simulink model "ex_pdcont"  (R2013a)
settings: Solver=ode1  StartTime=0.0  StopTime=inf  FixedStep=0.001  RelTol=1e-3
values from neighbouring files (symbols this model uses):
  kD = -0.399    [pdcont_data1.mat]    (also in pdcont_data2.mat = -0.022; pdcont_data3.mat = 0.261)
  kP = 7.075    [pdcont_data1.mat]    (also in pdcont_data2.mat; pdcont_data3.mat)
undefined symbols (not defined in the file or in its folder): HIL
libraries: quarc_library x3
settings Model: SimulationMode=external  ExtModeTrigDuration=500000  Creator=student  LastModifiedBy=student
settings SolverCC: PositivePriorityOrder=on
settings RTWCC: SystemTargetFile=quarc_win64.tlc  TemplateMakefile=quarc_default_tmf  Description=QUARC Win64 Target  ProcessScript=quarc_win64_make_rtw_hook
settings STFCustomTargetCC: TargetPreCompLibLocation=C:\PROGRA~3\QUARC\lib\2013a\win64\release  GeneratePreprocessorConditionals=Disable all  CombineOutputUpdateFcns=on  SystemTargetFile=quarc_win64.tlc
settings GRTTargetCC: TargetPreCompLibLocation=C:\PROGRA~3\QUARC\lib\2013a\win64\release  ParMdlRefBuildCompliant=off  CompOptLevelCompliant=off  ConcurrentExecutionCompliant=off  MatFileLogging=off  ExtMode=on  ExtModeMexFile=quarc_comm

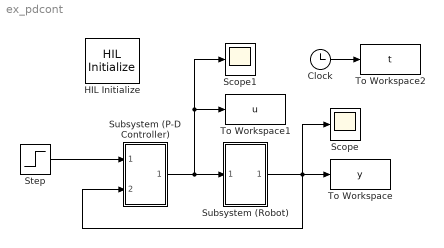
== system ex_pdcont ==
  Clock : Clock
  HIL Initialize : quarc_library/Data Acquisition/Generic/Configuration/HIL Initialize  Priority=-99  object_name=HIL-1  board_type=q8_usb  board_number=0  board_options=update_rate=normal;decimation=1  exclusive=off  active=off  hardware_clocks=[0:2]  clock_modes=[]  initial_clock_frequencies=[]  set_clock_params_at_start=off  set_clock_params_at_switch_in=off  set_clock_frequencies_at_start=off  set_clock_frequencies_at_switch_in=off  analog_input_channels=[0:7]  analog_input_maximums=5  analog_input_minimums=-5  set_analog_input_params_at_start=on  set_analog_input_params_at_switch_in=off  analog_output_channels=[0:7]  analog_output_maximums=10  analog_output_minimums=-10  initial_analog_outputs=[0]  final_analog_outputs=[0]  watchdog_analog_outputs=0  set_analog_output_params_at_start=on  set_analog_output_params_at_switch_in=off  set_analog_outputs_at_start=on  set_analog_outputs_at_switch_in=off  set_analog_outputs_at_terminate=on  set_analog_outputs_at_switch_out=off  set_analog_outputs_on_watchdog=off  digital_input_channels=[]  digital_output_channels=[]  digital_output_configuration=[]  initial_digital_outputs=[1]  final_digital_outputs=[1]  watchdog_digital_outputs=[1]  set_digital_output_params_at_start=off  set_digital_output_params_at_switch_in=off  set_digital_outputs_at_start=on  set_digital_outputs_at_switch_in=off  set_digital_outputs_at_terminate=on  set_digital_outputs_at_switch_out=off  set_digital_outputs_on_watchdog=off  encoder_channels=[0:7]  quadrature=[4]  encoder_filter_frequency=[]  initial_encoder_counts=[0]  set_encoder_params_at_start=on  set_encoder_params_at_switch_in=off  set_encoder_counts_at_start=on  set_encoder_counts_at_switch_in=off  pwm_channels=[0:7]  pwm_modes=0  pwm_frequency=99.532799999999995e6/4095  pwm_configuration=[0]  pwm_alignment=[0]  pwm_polarity=[1]  pwm_leading_deadband=[0]  pwm_trailing_deadband=[0]  initial_pwm_outputs=[0]  final_pwm_outputs=[0]  watchdog_pwm_outputs=[0]  set_pwm_params_at_start=on  set_pwm_params_at_switch_in=off  set_pwm_outputs_at_start=on  set_pwm_outputs_at_switch_in=off  set_pwm_outputs_at_terminate=on  set_pwm_outputs_at_switch_out=off  set_pwm_outputs_on_watchdog=off  other_output_channels=[]  initial_other_outputs=[]  final_other_outputs=[]  watchdog_other_outputs=[]  set_other_outputs_at_start=off  set_other_outputs_at_switch_in=off  set_other_outputs_at_terminate=off  set_other_outputs_at_switch_out=off  set_other_outputs_on_watchdog=off
  Scope : Scope
      settings: TimeRange=1  YMin=0  YMax=1.5
  Scope1 : Scope
      settings: TimeRange=1  YMax=10
  Step : Step  Time=0  After=0  SampleTime=0
  Subsystem (P-D Controller) : Subsystem
  Subsystem (Robot) : Subsystem
  To Workspace : ToWorkspace  VariableName=y  SampleTime=-1
  To Workspace1 : ToWorkspace  VariableName=u  SampleTime=-1
  To Workspace2 : ToWorkspace  VariableName=t  SampleTime=-1
  wires:
  Clock/1 -> To Workspace2/1
  Subsystem (P-D Controller)/1(Out1) -> To Workspace1/1, Scope1/1, Subsystem (Robot)/1(In1)
  Step/1 -> Subsystem (P-D Controller)/1(In1)
  Subsystem (Robot)/1(Out1) -> Subsystem (P-D Controller)/2(In2), Scope/1, To Workspace/1

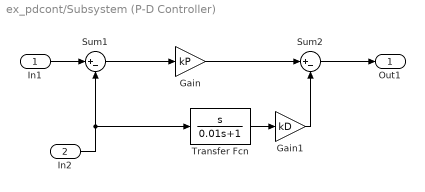
== system ex_pdcont/Subsystem (P-D Controller) ==
  In1 : Inport
  In2 : Inport  Port=2
  Gain : Gain  Gain=kP
  Gain1 : Gain  Gain=kD
  Sum1 : Sum  Inputs=|+-
  Sum2 : Sum  Inputs=|+-
  Transfer Fcn : TransferFcn  Numerator=[1 0]  Denominator=[0.01 1]
  Out1 : Outport
  wires:
  Sum1/1 -> Gain/1
  Sum2/1 -> Out1/1
  In1/1 -> Sum1/1
  Gain/1 -> Sum2/1
  Gain1/1 -> Sum2/2
  In2/1 -> Transfer Fcn/1, Sum1/2
  Transfer Fcn/1 -> Gain1/1

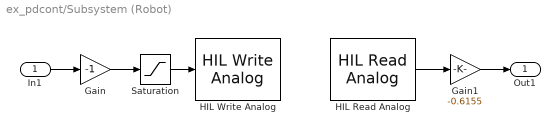
== system ex_pdcont/Subsystem (Robot) ==
  In1 : Inport
  Gain : Gain  Gain=-1
  Gain1 : Gain  Gain=-0.6155
  HIL Read Analog : quarc_library/Data Acquisition/Generic/Immediate I//O/HIL Read Analog  object_name=HIL-1  channels=1  sample_time=qc_get_step_size  active=on  vector_output=off
  HIL Write Analog : quarc_library/Data Acquisition/Generic/Immediate I//O/HIL Write Analog  object_name=HIL-1  channels=1  sample_time=-1  active=off  vector_input=off
  Saturation : Saturate  UpperLimit=10  LowerLimit=-10
  Out1 : Outport
  wires:
  HIL Read Analog/1 -> Gain1/1
  Saturation/1 -> HIL Write Analog/1
  Gain/1 -> Saturation/1
  In1/1 -> Gain/1
  Gain1/1 -> Out1/1
